simulink model "calcul_vitesse_roues"  (R2024b)
settings: Solver=FixedStepAuto  StartTime=0.0  StopTime=10.0  FixedStep=Ts  RelTol=1e-3
values from neighbouring files (symbols this model uses):
  J = 0.5    [main_data_vehicle.m]
  Re = 0.228    [main_data_vehicle.m]
  Ts = 0.001    [main_data_vehicle.m]
  v0 = 0.001    [main_data_vehicle.m]
settings Model: Creator=marti  LastModifiedBy=Filip

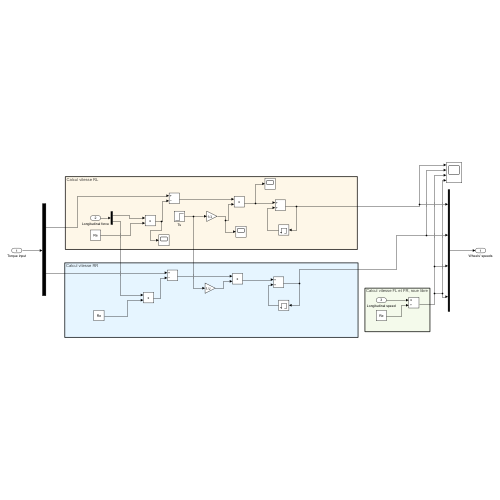
[thumbnail: Simulink's stored preview of the top-level diagram]
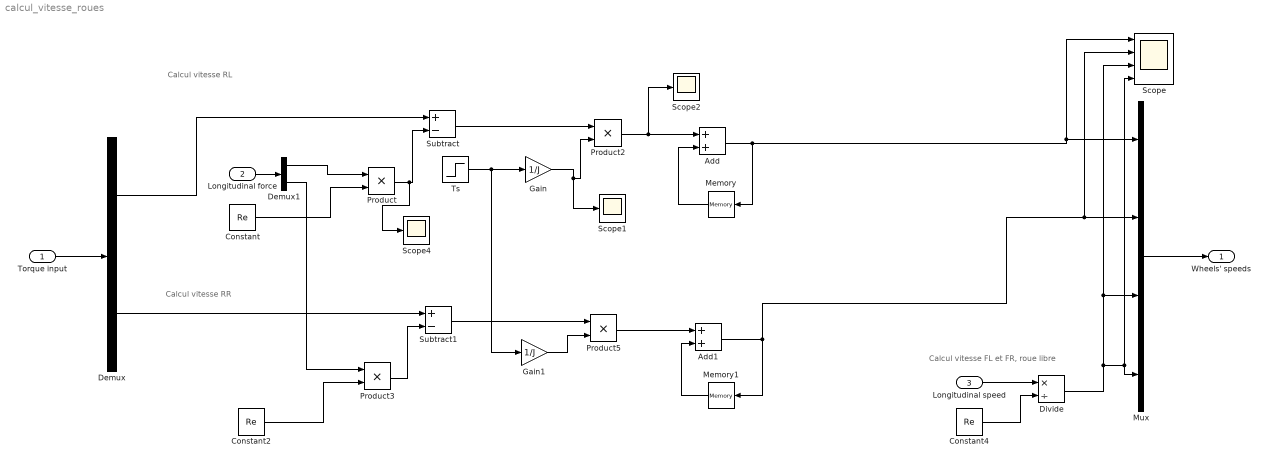
== system calcul_vitesse_roues ==
  note: Calcul vitesse FL et FR, roue libre
  note: Calcul vitesse RL
  note: Calcul vitesse RR
  Torque input : Inport
  Longitudinal force : Inport  Port=2
  Longitudinal speed : Inport  Port=3
  Add : Sum
  Add1 : Sum
  Constant : Constant  Value=Re
  Constant2 : Constant  Value=Re
  Constant4 : Constant  Value=Re
  Demux : Demux  Outputs=2
  Demux1 : Demux  Outputs=2
  Divide : Product  Inputs=*/
  Gain : Gain  Gain=1/J
  Gain1 : Gain  Gain=1/J
  Memory : Memory  InitialCondition=v0/Re
  Memory1 : Memory  InitialCondition=v0/Re
  Mux : Mux
  Product{,2..3,5} (4 alike) : Product
  Scope : Scope  NumInputPorts=4
  Scope1 : Scope
  Scope2 : Scope
  Scope4 : Scope
  Subtract : Sum  Inputs=+-
  Subtract1 : Sum  Inputs=+-
  Ts : Step  Time=0  After=Ts  SampleTime=0
  Wheels' speeds : Outport
  wires:
  Constant/1 -> Product/2
  Product/1 -> Scope4/1, Subtract/2
  Ts/1 -> Gain1/1, Gain/1
  Gain/1 -> Scope1/1, Product2/2
  Subtract/1 -> Product2/1
  Product2/1 -> Scope2/1, Add/1
  Add/1 -> Scope/1, Mux/1, Memory/1
  Memory/1 -> Add/2
  Torque input/1 -> Demux/1
  Subtract1/1 -> Product5/1
  Constant2/1 -> Product3/2
  Gain1/1 -> Product5/2
  Add1/1 -> Scope/2, Mux/2, Memory1/1
  Memory1/1 -> Add1/2
  Product3/1 -> Subtract1/2
  Product5/1 -> Add1/1
  Demux/2 -> Subtract1/1
  Demux/1 -> Subtract/1
  Longitudinal speed/1 -> Divide/1
  Constant4/1 -> Divide/2
  Divide/1 -> Scope/4, Mux/4, Scope/3, Mux/3
  Mux/1 -> Wheels' speeds/1
  Longitudinal force/1 -> Demux1/1
  Demux1/1 -> Product/1
  Demux1/2 -> Product3/1
